simulink model "vbyfcontrolpmsm_interrupt_2016a"  (R2016a)
settings: Solver=ode4  StartTime=0.0  StopTime=20  FixedStep=Ts  RelTol=1e-3
values from neighbouring files (symbols this model uses):
  Cdc = 100e-6    (= 0.0001)    [control_simulation_parameters.m]    (also in pmsm_vbyf_sim_parameters.m = 1.5e-05; vbyfcontrolim_sim.m)
  frated = 50    [vbyfcontrolim_sim.m]
  fsw = 10e3    (= 10000)    [control_simulation_parameters.m]    (also in pmsm_vbyf_sim_parameters.m; vbyfcontrolim_sim.m)
  phase = [0 90 0 90]    [control_simulation_parameters.m]    (also in pmsm_vbyf_sim_parameters.m = [0])
  Rin = 10    [control_simulation_parameters.m]    (also in pmsm_vbyf_sim_parameters.m = 1; vbyfcontrolim_sim.m = 1e-06)
  Tload = 30    [pmsm_vbyf_sim_parameters.m]    (also in vbyfcontrolim_sim.m = 10)
  Ts = 100e-9    (= 1e-07)    [control_simulation_parameters.m]    (also in pmsm_vbyf_sim_parameters.m = 1e-06; vbyfcontrolim_sim.m = 1e-06)
  VbyfFreqSteps = 2    [vbyfcontrolim_sim.m]
  VbyfStepTime = 0.2    [vbyfcontrolim_sim.m]
  Vin = Vdc + Rin*(Pout/Vdc)    (= 366.666666667)    [control_simulation_parameters.m]    (also in pmsm_vbyf_sim_parameters.m = 276.981317008; vbyfcontrolim_sim.m = 750)
  Vrated = Vllrated/sqrt(3)    [vbyfcontrolim_sim.m]
undefined symbols (not defined in the file or in its folder): Initial_freq, Lload, Rload, start_time, start_time_deceleration
libraries: powerlib x17, powerlib_meascontrol x3
settings Model: SimulationMode=accelerator  Creator=ugurm  LastModifiedBy=admin
settings DataIOCC: LimitDataPoints=on  SaveFormat=Array
settings DebuggingCC: UnderspecifiedInitializationDetection=Classic  MergeDetectMultiDrivingBlocksExec=none  SolverPrmCheckMsg=warning  StateNameClashWarn=warning
settings HardwareCC: ProdBitPerPointer=32  ProdLargestAtomicFloat=None  ProdIntDivRoundTo=Undefined  ProdEndianess=Unspecified  ProdWordSize=32  ProdHWDeviceType=32-bit Generic
settings ModelReferenceCC: PropagateSignalLabelsOutOfModel=off
settings SimscapeCC: SimscapeNormalizeSystem=off

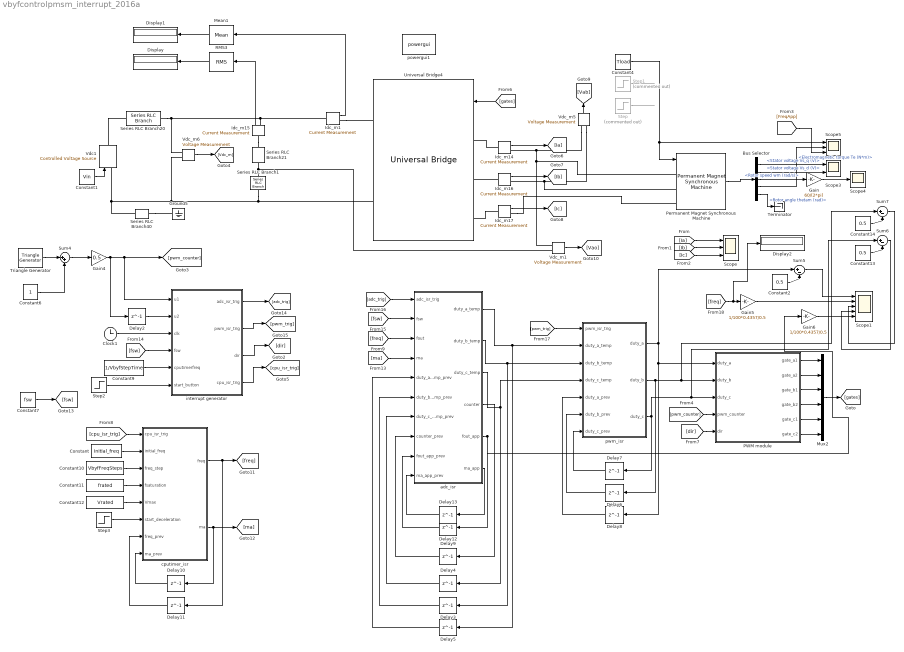
== system vbyfcontrolpmsm_interrupt_2016a ==
  Bus Selector : BusSelector  OutputSignals=Stator voltage Vs_q (V),Stator voltage Vs_d (V),Rotor speed wm (rad/s),Electromagnetic torque Te (N*m),Rotor angle thetam (rad)
  Clock1 : Clock
  Constant : Constant  Value=Initial_freq
  Constant1 : Constant  Value=Vin
  Constant10 : Constant  Value=VbyfFreqSteps
  Constant11 : Constant  Value=frated
  Constant12 : Constant  Value=Vrated
  Constant13 : Constant  Value=0.5
  Constant14 : Constant  Value=0.5
  Constant2 : Constant  Value=0.5
  Constant4 : Constant  Value=Tload
  Constant6 : Constant
  Constant7 : Constant  Value=fsw
  Constant9 : Constant  Value=1/VbyfStepTime
  Delay{2..13} (12 alike) : Delay  DelayLength=1
  Display : Display
  Display1 : Display
  Display2 : Display
  Gain : Gain  Gain=60/(2*pi)
  Gain4 : Gain  Gain=0.5
  Gain5 : Gain  Gain=1/100*0.4357/0.5
  Gain6 : Gain  Gain=1/100*0.4357/0.5
  Ground5 : powerlib/Elements/Ground  LConnTagsString=a
  Idc_m{1,14..17} (5 alike) : powerlib/Measurements/Current Measurement  PhasorSimulation=off  OutputType=Complex  PSBequivalent=0
  Mean1 : powerlib_meascontrol/Measurements/Mean  Freq=fout  Vinit=0  Ts=0
  Mux2 : Mux  Inputs=6
  PWM module : MATLAB Function  TreatAsAtomicUnit=on
  Permanent Magnet Synchronous Machine : powerlib/Machines/Permanent Magnet Synchronous Machine  NbPhases=3  FluxDistribution=Sinusoidal  RotorType=Salient-pole  MechanicalLoad=Torque Tm  PresetModel=No  ShowDetailedParameters=on  MeasurementBus=off  Resistance=0.320  Inductance=8.5e-3  dqInductances=[3.1e-3,3.6e-3]  La=0.000395  MachineConstant=Flux linkage established by magnets (V.s)  Flux=0.18  VoltageCst=326.4839  TorqueCst=2.7  Flat=120  Mechanical=[0.0027 0.0004924 10 0]  PolePairs=4  InitialConditions=[0,0, 0,0]  InitialConditions5ph=[0 0 0 0 0 0]  TsPowergui=0  TsBlock=-1  RefAngle=90 degrees behind phase A axis (modified Park)
  RMS3 : powerlib_meascontrol/Measurements/RMS  TrueRMS=on  Freq=fout  RMSInit=0  Ts=0
  Scope : Scope  NumInputPorts=3
  Scope1 : Scope  NumInputPorts=5
  Scope3 : Scope  NumInputPorts=2
  Scope4 : Scope
  Scope5 : Scope  NumInputPorts=3
  Series RLC Branch1 : powerlib/Elements/Series RLC Branch  LConnTagsString=__new0  RConnTagsString=__new0  BranchType=C  Resistance=Rload  Inductance=Lload  SetiL0=off  InitialCurrent=0  Capacitance=Cdc*2  Setx0=off  InitialVoltage=0  Measurements=None
  Series RLC Branch20 : powerlib/Elements/Series RLC Branch  LConnTagsString=__new0  RConnTagsString=__new0  BranchType=R  Resistance=Rin  Inductance=Lload  SetiL0=off  InitialCurrent=0  Capacitance=1e-6  Setx0=off  InitialVoltage=0  Measurements=None
  Series RLC Branch21 : powerlib/Elements/Series RLC Branch  LConnTagsString=__new0  RConnTagsString=__new0  BranchType=C  Resistance=Rload  Inductance=Lload  SetiL0=off  InitialCurrent=0  Capacitance=Cdc*2  Setx0=off  InitialVoltage=0  Measurements=None
  Series RLC Branch40 : powerlib/Elements/Series RLC Branch  LConnTagsString=__new0  RConnTagsString=__new0  BranchType=R  Resistance=1e12  Inductance=Lload  SetiL0=off  InitialCurrent=0  Capacitance=1e-6  Setx0=off  InitialVoltage=0  Measurements=None
  Step : Step  Commented=on  Time=7  After=Tload  SampleTime=0
  Step1 : Step  Commented=on  Time=6  After=Tload  SampleTime=0
  Step2 : Step  Time=start_time  SampleTime=0
  Step3 : Step  Time=start_time_deceleration  SampleTime=0
  Sum4 : Sum  Inputs=|++
  Sum5 : Sum  Inputs=|+-
  Sum6 : Sum  Inputs=|+-
  Sum7 : Sum  Inputs=|+-
  Terminator : Terminator
  Triangle Generator : powerlib_meascontrol/Pulse & Signal Generators/Triangle Generator  Freq=fsw  Phase=0  Ts=0
  Universal Bridge4 : powerlib/Power Electronics/Universal Bridge  Arms=3  SnubberResistance=1e5  SnubberCapacitance=inf  Device=IGBT / Diodes  Ron=1e-6  Lon=0  ForwardVoltages="[  0  0  ]"  ForwardVoltage=0  GTOparameters=[ 10e-6 , 20e-6 ]  IGBTparameters=[0,0]  Measurements=None  Measurements_2=None  converterType=Rectifier
  Vdc1 : powerlib/Electrical Sources/Controlled Voltage Source  Initialize=off  Source_Type=DC  Amplitude=200  Phase=0  Frequency=0  Measurements=None
  Vdc_m1 : powerlib/Measurements/Voltage Measurement  PhasorSimulation=off  OutputType=Complex  PSBequivalent=0
  Vdc_m5 : powerlib/Measurements/Voltage Measurement  PhasorSimulation=off  OutputType=Complex  PSBequivalent=0
  Vdc_m6 : powerlib/Measurements/Voltage Measurement  PhasorSimulation=off  OutputType=Complex  PSBequivalent=0
  adc_isr : MATLAB Function  TreatAsAtomicUnit=on
  cputimer_isr : MATLAB Function  TreatAsAtomicUnit=on
  interrupt generator : MATLAB Function  TreatAsAtomicUnit=on
  powergui1 : powerlib/powergui  Priority=1  SimulationMode=Discrete  SampleTime=Ts  frequency=60  Iterations=50  frequencyindice=0  Pbase=100e6  ErrMax=1e-4  UnitsV=kV  UnitsW=MW  buscounter=0  FunctionMessages=off  echomessages=off  EnableUseOfTLC=off  CurrentSourceSwitches=off  DisableSnubberDevices=off  DisableRonSwitches=off  DisableVfSwitches=off  DisplayEquations=off  AutomaticDiscreteSolvers=off  SolverType=Tustin  Interpol=off  ExternalGateDelay=off  methode=off  Ts=0  x0status=blocks  SPID=off  SwTol=0  HookPort=off  NonlinearTolerance=0  nMaxIteration=15  ContinueOnMaxIteration=off  RestoreLinks=warning  ResistiveCurrentMeasurement=off  Frange=[0:2:500]  Ylog=off  Xlog=on  ShowGrid=off  save=off  variable=ZData  structure=Vdc  ZoomFFT=off  StartTime=0.04  cycles=5  DisplayStyle=5  fundamental=50  FreqAxis=off  MaxFrequency=30000  frequencyindicesteady=1  RmsSteady=1  display=off
  pwm_isr : MATLAB Function  TreatAsAtomicUnit=on
  wires:
  Constant1/1 -> Vdc1/1
  Idc_m15/1 -> RMS3/1
  Vdc_m6/1 -> [Vdc_m]
  RMS3/1 -> Display/1
  Idc_m1/1 -> Mean1/1
  Mean1/1 -> Display1/1
  Idc_m14/1 -> [Ia]
  Idc_m16/1 -> [Ib]
  Idc_m17/1 -> [Ic]
  Vdc_m5/1 -> [Vab]
  Vdc_m1/1 -> [Vao]
  [Ia] -> Scope/1
  [Ic] -> Scope/3
  [Ib] -> Scope/2
  Permanent Magnet Synchronous Machine/1 -> Bus Selector/1
  Bus Selector/1 -> Scope3/1  "<Stator voltage Vs_q (V)>"
  Bus Selector/2 -> Scope3/2  "<Stator voltage Vs_d (V)>"
  Bus Selector/3 -> Gain/1  "<Rotor speed wm (rad/s)>"
  Bus Selector/4 -> Scope5/2  "<Electromagnetic torque Te (N*m)>"
  Bus Selector/5 -> Terminator/1  "<Rotor angle thetam (rad)>"
  Gain/1 -> Scope4/1
  [FreqApp] -> Scope5/3
  Constant4/1 -> Scope5/1, Permanent Magnet Synchronous Machine/1
  Triangle Generator/1 -> Sum4/1
  Constant6/1 -> Sum4/2
  Sum4/1 -> Gain4/1
  Gain4/1 -> [pwm_counter], interrupt generator/1(u1), Delay2/1
  Delay2/1 -> interrupt generator/2(u2)
  Clock1/1 -> interrupt generator/3(clk)
  adc_isr/1(duty_a_temp) -> Delay5/1, pwm_isr/2(duty_a_temp)
  adc_isr/2(duty_b_temp) -> Delay3/1, pwm_isr/3(duty_b_temp)
  adc_isr/3(duty_c_temp) -> pwm_isr/4(duty_c_temp), Delay4/1
  [pwm_counter] -> PWM module/4(pwm_counter)
  PWM module/6(gate_c2) -> Mux2/6
  PWM module/4(gate_b2) -> Mux2/4
  PWM module/5(gate_c1) -> Mux2/5
  PWM module/3(gate_b1) -> Mux2/3
  PWM module/2(gate_a2) -> Mux2/2
  PWM module/1(gate_a1) -> Mux2/1
  [gates] -> Universal Bridge4/1
  Mux2/1 -> [gates]
  [dir] -> PWM module/5(dir)
  interrupt generator/3(dir) -> [dir]
  Delay5/1 -> adc_isr/5(duty_a_temp_prev)
  Delay3/1 -> adc_isr/6(duty_b_temp_prev)
  Delay4/1 -> adc_isr/7(duty_c_temp_prev)
  Delay7/1 -> pwm_isr/7(duty_c_prev)
  Delay6/1 -> pwm_isr/6(duty_b_prev)
  Delay8/1 -> pwm_isr/5(duty_a_prev)
  pwm_isr/3(duty_c) -> Delay7/1, Sum6/1, PWM module/3(duty_c)
  pwm_isr/1(duty_a) -> Sum5/1, PWM module/1(duty_a), Delay8/1
  [fsw] -> interrupt generator/4(fsw)
  [freq] -> adc_isr/3(fout)
  Delay9/1 -> adc_isr/8(counter_prev)
  Constant9/1 -> interrupt generator/5(cputimerfreq)
  Constant/1 -> cputimer_isr/2(initial_freq)
  interrupt generator/4(cpu_isr_trig) -> [cpu_isr_trig]
  [cpu_isr_trig] -> cputimer_isr/1(cpu_isr_trig)
  Constant10/1 -> cputimer_isr/3(freq_step)
  Constant11/1 -> cputimer_isr/4(fsaturation)
  Constant12/1 -> cputimer_isr/5(Vmax)
  cputimer_isr/2(ma) -> [ma], Delay10/1
  Delay10/1 -> cputimer_isr/8(ma_prev)
  cputimer_isr/1(freq) -> [freq], Delay11/1
  Delay11/1 -> cputimer_isr/7(freq_prev)
  [ma] -> adc_isr/4(ma)
  Constant7/1 -> [fsw]
  [fsw] -> adc_isr/2(fsw)
  interrupt generator/1(adc_isr_trig) -> [adc_trig]
  [adc_trig] -> adc_isr/1(adc_isr_trig)
  interrupt generator/2(pwm_isr_trig) -> [pwm_trig]
  [pwm_trig] -> pwm_isr/1(pwm_isr_trig)
  adc_isr/5(fout_app) -> Gain6/1, Delay12/1
  adc_isr/6(ma_app) -> Delay13/1
  Delay13/1 -> adc_isr/10(ma_app_prev)
  Delay12/1 -> adc_isr/9(fout_app_prev)
  Gain5/1 -> Scope1/2
  [freq] -> Display2/1, Gain5/1
  adc_isr/4(counter) -> Delay9/1
  Constant2/1 -> Sum5/2
  Sum5/1 -> Scope1/1
  Constant13/1 -> Sum6/2
  Constant14/1 -> Sum7/2
  pwm_isr/2(duty_b) -> Sum7/1, PWM module/2(duty_b), Delay6/1
  Sum7/1 -> Scope1/3
  Sum6/1 -> Scope1/4
  Gain6/1 -> Scope1/5
  Step2/1 -> interrupt generator/6(start_button)
  Step3/1 -> cputimer_isr/6(start_deceleration)
  Step/1 -> ?
  Step1/1 -> ?
  connections:
  Vdc_m5/LConn1 -- Permanent Magnet Synchronous Machine/LConn1 -- Vdc_m1/LConn1 -- Idc_m14/RConn1
  Universal Bridge4/RConn2 -- Vdc_m6/LConn2 -- Vdc1/LConn1 -- Series RLC Branch40/LConn1 -- Series RLC Branch1/RConn1
  Series RLC Branch40/RConn1 -- Ground5/LConn1
  Idc_m14/LConn1 -- Universal Bridge4/LConn1
  Idc_m15/LConn1 -- Series RLC Branch21/LConn1
  Vdc1/RConn1 -- Series RLC Branch20/LConn1
  Idc_m16/LConn1 -- Universal Bridge4/LConn2
  Idc_m17/LConn1 -- Universal Bridge4/LConn3
  Vdc_m5/LConn2 -- Permanent Magnet Synchronous Machine/LConn2 -- Idc_m16/RConn1
  Idc_m1/RConn1 -- Universal Bridge4/RConn1
  Idc_m1/LConn1 -- Series RLC Branch20/RConn1 -- Vdc_m6/LConn1 -- Idc_m15/RConn1
  Series RLC Branch1/LConn1 -- Vdc_m1/LConn2 -- Series RLC Branch21/RConn1
  Idc_m17/RConn1 -- Permanent Magnet Synchronous Machine/LConn3

== matlab function vbyfcontrolpmsm_interrupt_2016a/adc_isr ==
  data: adc_isr_trig input; fsw input; fout input; ma input; duty_a_temp_prev input; duty_b_temp_prev input; duty_c_temp_prev input; counter_prev input; duty_a_temp output; duty_b_temp output; duty_c_temp output; counter output; fout_app_prev input; ma_app_prev input; fout_app output; ma_app output
function [duty_a_temp,duty_b_temp,duty_c_temp,counter,fout_app,ma_app] = fcn(adc_isr_trig,...
    fsw,fout,ma,duty_a_temp_prev,duty_b_temp_prev,duty_c_temp_prev,counter_prev,fout_app_prev,ma_app_prev)

if (adc_isr_trig == 1) % interrupt on zero event
    counter = counter_prev+1;
    fout_app = fout_app_prev;
    if(counter > (fsw/fout_app)-1)
        counter = 0;
        fout_app = fout;
        ma_app = ma;
    else
        fout_app = fout_app_prev;
        ma_app = ma_app_prev;
    end
    duty_a_temp = (ma_app*sin(2*pi*fout_app*counter/fsw)+1)/2;
    duty_b_temp = (ma_app*sin(2*pi*fout_app*counter/fsw-2*pi/3)+1)/2;
    duty_c_temp = (ma_app*sin(2*pi*fout_app*counter/fsw+2*pi/3)+1)/2;
else
    duty_a_temp = duty_a_temp_prev;
    duty_b_temp = duty_b_temp_prev;
    duty_c_temp = duty_c_temp_prev;
    counter = counter_prev;
    %fout_app = fout_app_prev;
    %ma_app = ma_app_prev;
    if (fout_app_prev == 0)
       ma_app = ma;
       fout_app = fout;
    else
        ma_app = ma_app_prev;
        fout_app = fout_app_prev;
    end
end;

== matlab function vbyfcontrolpmsm_interrupt_2016a/pwm_isr ==
  data: duty_a output; pwm_isr_trig input; duty_a_temp input; duty_b_temp input; duty_c_temp input; duty_b output; duty_c output; duty_a_prev input; duty_b_prev input; duty_c_prev input
function [duty_a,duty_b,duty_c] = fcn(pwm_isr_trig,...
    duty_a_temp,duty_b_temp,duty_c_temp,duty_a_prev,duty_b_prev,duty_c_prev)

if (pwm_isr_trig == 1) % interrupt on prd event
    duty_a = duty_a_temp;
    duty_b = duty_b_temp;
    duty_c = duty_c_temp;
else
    duty_a = duty_a_prev;
    duty_b = duty_b_prev;
    duty_c = duty_c_prev;
end;

== matlab function vbyfcontrolpmsm_interrupt_2016a/interrupt generator ==
  data: u1 input; adc_isr_trig output; u2 input; clk input; pwm_isr_trig output; dir output; fsw input; cputimerfreq input; cpu_isr_trig output; start_button input
function [adc_isr_trig,pwm_isr_trig,dir,cpu_isr_trig] = fcn(u1,u2,clk,fsw,...
    cputimerfreq,start_button)

if (rem(clk,1/fsw) == 0)
    adc_isr_trig = 1; % interrupt on zero
    dir = 0;
else
    adc_isr_trig = 0;
    if (u1 > u2)
        dir = 1; % up
    else
        dir = 0; % down
    end;
end;

if (rem(clk*2,1/fsw) == 0 && rem(clk,1/fsw) ~= 0)
    pwm_isr_trig = 1; % interrupt on period
else
    pwm_isr_trig = 0;
end;

if (start_button)
    if (rem(clk,1/cputimerfreq) == 0)
        cpu_isr_trig = 1;
    else
        cpu_isr_trig = 0;
    end
else
    cpu_isr_trig = 0;
end

== matlab function vbyfcontrolpmsm_interrupt_2016a/PWM module ==
  data: duty_a input; gate_a1 output; duty_b input; duty_c input; gate_a2 output; gate_b1 output; gate_b2 output; gate_c1 output; gate_c2 output; pwm_counter input; dir input
function [gate_a1,gate_a2,gate_b1,gate_b2,gate_c1,gate_c2] = fcn(duty_a,duty_b,duty_c,pwm_counter,dir)

if (duty_a > pwm_counter)
    gate_a1 = 1;
    gate_a2 = 0;
else
    gate_a1 = 0;
    gate_a2 = 1;
end;
if (duty_b > pwm_counter)
    gate_b1 = 1;
    gate_b2 = 0;
else
    gate_b1 = 0;
    gate_b2 = 1;
end;
if (duty_c > pwm_counter)
    gate_c1 = 1;
    gate_c2 = 0;
else
    gate_c1 = 0;
    gate_c2 = 1;
end;

== matlab function vbyfcontrolpmsm_interrupt_2016a/cputimer_isr ==
  data: cpu_isr_trig input; initial_freq input; freq_step input; fsaturation input; Vmax input; start_deceleration input; freq output; ma output; freq_prev input; ma_prev input
function [freq,ma] = fcn(cpu_isr_trig,initial_freq,freq_step,...
    fsaturation,Vmax,start_deceleration,freq_prev,ma_prev)

if (cpu_isr_trig == 1) % interrupt on cputimer event
    if (start_deceleration == 0)
        if (freq_prev + freq_step) > fsaturation
            freq = fsaturation;
        elseif (freq_prev < initial_freq)
            freq = freq_prev + initial_freq;
        else
            freq = freq_prev + freq_step;
        end
    else
        if (freq_prev - freq_step) < 0
            freq = 0;
        else
            freq = freq_prev - freq_step;
        end
    end
    ma = freq*(Vmax/fsaturation)*(sqrt(3)/(750*0.612));
else
    %     if (freq_prev == 0)
    %        freq = initial_freq;
    %     else
    %         freq = freq_prev;
    %     end
    freq = freq_prev;
    ma = ma_prev;
end;
